simulink model "EE238BuckCon"  (R2018a)
settings: Solver=VariableStepAuto  StartTime=0.0  StopTime=0.008  MaxStep=1e-4  RelTol=1e-4  EnableMultiTasking=on
libraries: powerlib x13, powerlib_meascontrol x1
Description:
  | Copyright 2008-2018 The MathWorks, Inc.
settings Model: Creator=MathWorks  LastModifiedBy=Kishore Chatterjee
settings SolverCC: SolverResetMethod=Robust
settings OptimizationCC: EfficientFloat2IntCast=on  LifeSpan=inf
settings DebuggingCC: UniqueDataStoreMsg=error  StrictBusMsg=ErrorOnBusTreatedAsVector  SFUnexpectedBacktrackingDiag=warning  SFNoUnconditionalDefaultTransitionDiag=warning  SFExecutionAtInitializationDiag=none
settings CodeAppCC: StateflowObjectComments=on
settings GRTTargetCC: TargetLangStandard=C89/C90 (ANSI)  GeneratePreprocessorConditionals=Disable all
settings ConfigComp: CovMetricSettings=dw  CovHtmlReporting=on  CovSaveCumulativeToWorkspaceVar=on  CovSaveSingleToWorkspaceVar=on  CovExternalEMLEnable=off
settings SimscapeCC: SimscapeNormalizeSystem=off  SimscapeNominalValues={1, 'bar'; 1, 'cm^3/s'; 1, 'bar*kg/s'; 1, 'kJ/kg'; 1, 'kW'; }

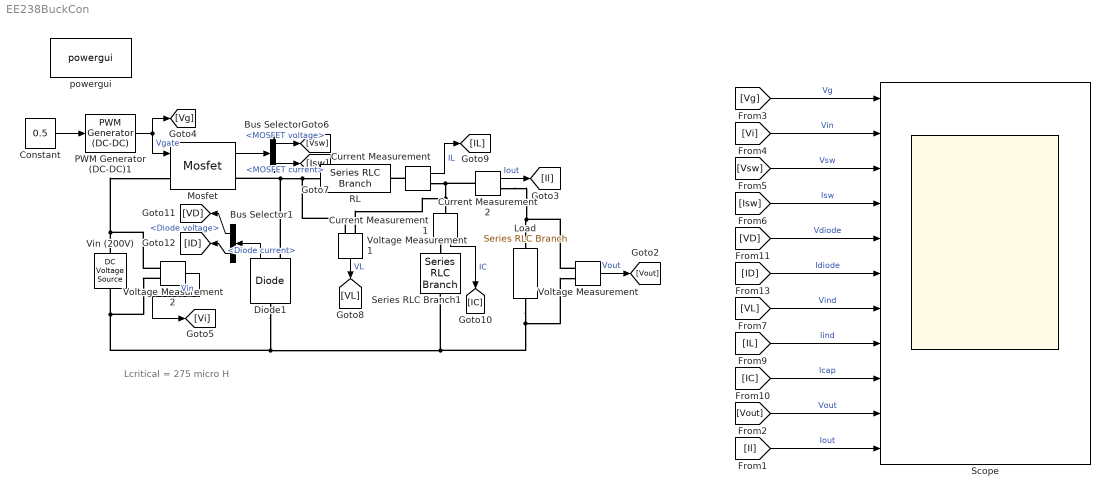
== system EE238BuckCon ==
  note: Lcritical = 275 micro H
  Bus Selector : BusSelector  OutputSignals=MOSFET voltage,MOSFET current
  Bus Selector1 : BusSelector  OutputSignals=Diode voltage,Diode current
  Constant : Constant  Value=0.5
  Current Measurement : powerlib/Measurements/Current Measurement  PhasorSimulation=off  OutputType=Complex  PSBequivalent=0
  Current Measurement1 : powerlib/Measurements/Current Measurement  PhasorSimulation=off  OutputType=Complex  PSBequivalent=0
  Current Measurement2 : powerlib/Measurements/Current Measurement  PhasorSimulation=off  OutputType=Complex  PSBequivalent=0
  Diode1 : powerlib/Power Electronics/Diode  Ron=1e-3  Lon=0  Vf=0  IC=0  UseSnubber=off  Rs=inf  Cs=inf  Measurements=on
  Load : powerlib/Elements/Series RLC Branch  LConnTagsString=__new0  RConnTagsString=__new0  BranchType=R  Resistance=100  Inductance=200e-6  SetiL0=off  InitialCurrent=0  Capacitance=400e-6  Setx0=off  InitialVoltage=0  Measurements=None
  Mosfet : powerlib/Power Electronics/Mosfet  Ron=1e-3  Lon=0  Rd=1e-3  Vfd=0  IC=0  Rs=inf  Cs=inf  Measurements=on
  PWM Generator (DC-DC)1 : powerlib_meascontrol/Pulse & Signal Generators/PWM Generator (DC-DC)  Fsw=5000  Ts=0
  RL : powerlib/Elements/Series RLC Branch  LConnTagsString=__new0  RConnTagsString=__new0  BranchType=RL  Resistance=0.02  Inductance=3e-3  SetiL0=off  InitialCurrent=0  Capacitance=1e-6  Setx0=off  InitialVoltage=0  Measurements=None
  Scope : Scope  NumInputPorts=11
  Series RLC Branch1 : powerlib/Elements/Series RLC Branch  LConnTagsString=__new0  RConnTagsString=__new0  BranchType=C  Resistance=1e-4  Inductance=200e-6  SetiL0=off  InitialCurrent=0  Capacitance=30e-6  Setx0=off  InitialVoltage=150  Measurements=None
  Vin (200V) : powerlib/Electrical Sources/DC Voltage Source  Amplitude=200  Measurements=None
  Voltage Measurement : powerlib/Measurements/Voltage Measurement  PhasorSimulation=off  OutputType=Complex  PSBequivalent=0
  Voltage Measurement1 : powerlib/Measurements/Voltage Measurement  PhasorSimulation=off  OutputType=Complex  PSBequivalent=0
  Voltage Measurement2 : powerlib/Measurements/Voltage Measurement  PhasorSimulation=off  OutputType=Complex  PSBequivalent=0
  powergui : powerlib/powergui  Priority=1  SimulationMode=Continuous  SampleTime=50e-6  frequency=60  Iterations=50  frequencyindice=0  Pbase=100e6  ErrMax=1e-4  UnitsV=kV  UnitsW=MW  buscounter=0  FunctionMessages=off  echomessages=off  EnableUseOfTLC=off  CurrentSourceSwitches=off  DisableSnubberDevices=off  DisableRonSwitches=off  DisableVfSwitches=off  DisplayEquations=off  SolverType=Tustin/Backward Euler (TBE)  Interpol=off  ExternalGateDelay=off  methode=off  Ts=100  x0status=blocks  SPID=on  SwTol=0  HookPort=off  RestoreLinks=warning  ResistiveCurrentMeasurement=off  Frange=[0:2:500]  Ylog=off  Xlog=on  ShowGrid=off  save=off  variable=ZData  structure=0  ZoomFFT=off  StartTime=0.0  cycles=1  DisplayStyle=1  fundamental=60  FreqAxis=off  MaxFrequency=1000  frequencyindicesteady=1  RmsSteady=1  display=off
  wires:
  Voltage Measurement/1 -> [Vout]  "Vout"
  PWM Generator (DC-DC)1/1 -> [Vg], Mosfet/1  "Vgate"
  Constant/1 -> PWM Generator (DC-DC)1/1
  Mosfet/1 -> Bus Selector/1
  Diode1/1 -> Bus Selector1/1
  Current Measurement2/1 -> [Il]  "Iout"
  [Il] -> Scope/11  "Iout"
  [Vout] -> Scope/10  "Vout"
  [Vg] -> Scope/1  "Vg"
  Voltage Measurement2/1 -> [Vi]  "Vin"
  [Vi] -> Scope/2  "Vin"
  Bus Selector/1 -> [Vsw]  "<MOSFET voltage>"
  [Vsw] -> Scope/3  "Vsw"
  Bus Selector/2 -> [Isw]  "<MOSFET current>"
  [Isw] -> Scope/4  "Isw"
  Voltage Measurement1/1 -> [VL]  "VL"
  [VL] -> Scope/7  "Vind"
  Current Measurement/1 -> [IL]  "IL"
  [IL] -> Scope/8  "Iind"
  Current Measurement1/1 -> [IC]  "IC"
  [IC] -> Scope/9  "Icap"
  Bus Selector1/1 -> [VD]  "<Diode voltage>"
  Bus Selector1/2 -> [ID]  "<Diode current>"
  [VD] -> Scope/5  "Vdiode"
  [ID] -> Scope/6  "Idiode"
  connections:
  Load/RConn1 -- Voltage Measurement2/LConn2 -- Vin (200V)/LConn1 -- Diode1/LConn1 -- Series RLC Branch1/RConn1 -- Voltage Measurement/LConn2
  Current Measurement/RConn1 -- Current Measurement2/LConn1 -- Voltage Measurement1/LConn1 -- Current Measurement1/LConn1
  Vin (200V)/RConn1 -- Voltage Measurement2/LConn1 -- Mosfet/LConn1
  Diode1/RConn1 -- Voltage Measurement1/LConn2 -- RL/LConn1 -- Mosfet/RConn1
  Current Measurement/LConn1 -- RL/RConn1
  Current Measurement1/RConn1 -- Series RLC Branch1/LConn1
  Voltage Measurement/LConn1 -- Current Measurement2/RConn1 -- Load/LConn1
